simulink model "leastsquarespolyfit_ref"  (Simulink 5.0)
settings: Solver=FixedStepDiscrete  StartTime=0.0  StopTime=10.0  RelTol=1e-3
libraries: dspsrcs4 x2, dsppolyfun x2
settings Model: Creator=ckamachi  LastModifiedBy=ckamachi  BlockReductionOpt=off  BooleanDataType=off

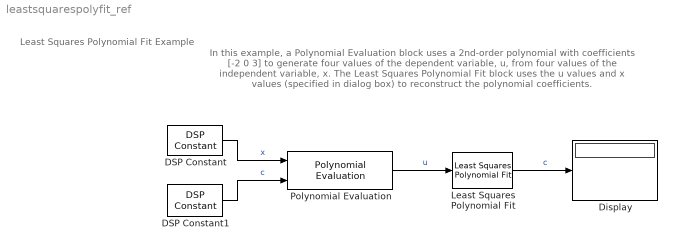
== system leastsquarespolyfit_ref ==
  note: Least Squares Polynomial Fit Example
  note: In this example, a Polynomial Evaluation block uses a 2nd-order
      | polynomial with coefficients [-2 0 3] to generate four values of
      | the dependent variable, u, from four values of the independent
      | variable, x. The Least Squares Polynomial Fit block uses the u
      | values and x values (specified in dialog box) to reconstruct the
      | polynomial coefficients.
  DSP Constant : dspsrcs4/DSP Constant  Value=[0:31]'/31  SampleMode=Discrete  discreteOutput=Sample-based  continuousOutput=Sample-based  sampTime=1  framePeriod=1  dataType=Inherit from 'Constant value'  wordLen=16  udDataType=sfix(16)  fracBitsMode=Best precision  numFracBits=15  InterpretAs1D=off  Ts=1  FramebasedOutput=off
  DSP Constant1 : dspsrcs4/DSP Constant  Value=[-2 0 3]'  SampleMode=Discrete  discreteOutput=Sample-based  continuousOutput=Sample-based  sampTime=1  framePeriod=1  dataType=Inherit from 'Constant value'  wordLen=16  udDataType=sfix(16)  fracBitsMode=Best precision  numFracBits=15  InterpretAs1D=off  Ts=1  FramebasedOutput=off
  Display : Display
  Least Squares Polynomial Fit : dsppolyfun/Least Squares Polynomial Fit  X=(0:31) / 31  N=2
  Polynomial Evaluation : dsppolyfun/Polynomial Evaluation  useConstCoeffs=off  constCoeffs=[5 4 3 2 1]
  wires:
  DSP Constant/1 -> Polynomial Evaluation/1  "x"
  Polynomial Evaluation/1 -> Least Squares Polynomial Fit/1  "u"
  Least Squares Polynomial Fit/1 -> Display/1  "c"
  DSP Constant1/1 -> Polynomial Evaluation/2  "c"
